simulink model "Bibliotheque"  (R2015a)
settings: Solver=ode45  StartTime=0.0  StopTime=10.0  RelTol=1e-3
undefined symbols (not defined in the file): B, D, dt, fv, gain_accelero, gain_effort_ext, gain_encodeur_moteur_rad, gain_intensite_moteur, gain_joy_X, gain_regle_mg, gain_tension_moteur, gain_vitesse_mm_s, gain_vitesse_tr_min, I, kprim, L, meq, National_Instruments, offset_effort_ext, offset_joy_X, offset_joy_Y, P, PCIe, r, sigbuilder_block, vecteur_de_tensions, vecteur_des_distances, Vsat
libraries: sldrtlib x35, simulink x4
settings Model: CovSFcnEnable=off  Creator=user  LastModifiedBy=ASUS
settings DataIOCC: SignalLoggingSaveFormat=ModelDataLogs
settings OptimizationCC: ExpressionDepthLimit=2147483647
settings DebuggingCC: UnderspecifiedInitializationDetection=Classic  MergeDetectMultiDrivingBlocksExec=none  SolverPrmCheckMsg=warning  FcnCallInpInsideContextMsg=EnableAllAsWarning  StateNameClashWarn=warning
settings GRTTargetCC: CombineOutputUpdateFcns=off  GRTInterface=on

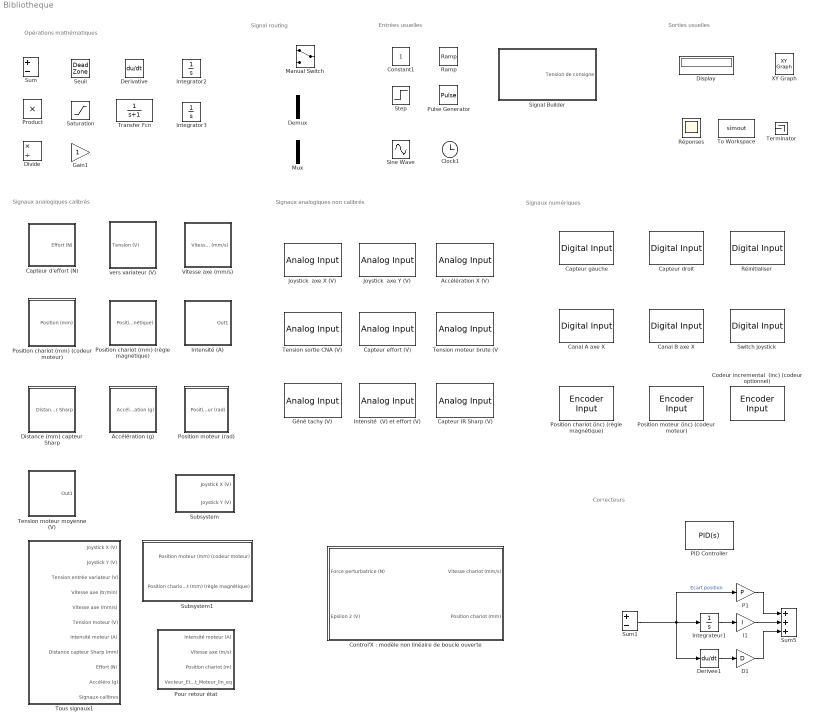
== system Bibliotheque ==
  note: Signaux numériques
  note: Signaux analogiques non calibrés
  note: Signaux analogiques calibrés
  note: Opérations mathématiques
  note: Signal routing
  note: Sorties usuelles
  note: Entrées usuelles
  note: Correcteurs
  Accélération (g) : Subsystem
      mask Display: image(imread('carte.jpg'))
  Accélération X (V) : sldrtlib/Analog Input  SampleTime=dt  MaxMissedTicks=10  ShowMissedTicks=off  YieldWhenWaiting=off  DrvName=National_Instruments/PCIe-6321  DrvAddress=4294967295  DrvOptions=[0 0 0 2 2 2 0]  Channels=15  RangeMode=1  VoltRange=1  DataType=1
      settings: AttributesFormatString=National Instruments\nPCIe-6321 [auto]
  Canal A axe X : sldrtlib/Digital Input  SampleTime=dt  MaxMissedTicks=10  ShowMissedTicks=off  YieldWhenWaiting=on  DrvName=National_Instruments/PCIe-6321  DrvAddress=4294967295  DrvOptions=[0 0 0 2 2 2 0]  Channels=5  BitMode=1  DataType=1
      settings: AttributesFormatString=National Instruments\nPCIe-6321 [auto]
  Canal B axe X : sldrtlib/Digital Input  SampleTime=dt  MaxMissedTicks=10  ShowMissedTicks=off  YieldWhenWaiting=on  DrvName=National_Instruments/PCIe-6321  DrvAddress=4294967295  DrvOptions=[0 0 0 2 2 2 0]  Channels=4  BitMode=1  DataType=1
      settings: AttributesFormatString=National Instruments\nPCIe-6321 [auto]
  Capteur IR Sharp (V) : sldrtlib/Analog Input  SampleTime=dt  MaxMissedTicks=10  ShowMissedTicks=off  YieldWhenWaiting=off  DrvName=National_Instruments/PCIe-6321  DrvAddress=4294967295  DrvOptions=[0 0 0 2 2 2 0]  Channels=7  RangeMode=1  VoltRange=1  DataType=1
      settings: AttributesFormatString=National Instruments\nPCIe-6321 [auto]
  Capteur d'effort (N) : Subsystem
      mask Display: image(imread('carte.jpg'))
  Capteur droit : sldrtlib/Digital Input  SampleTime=dt  MaxMissedTicks=10  ShowMissedTicks=off  YieldWhenWaiting=on  DrvName=National_Instruments/PCIe-6321  DrvAddress=4294967295  DrvOptions=[0 0 0 2 2 2 0]  Channels=2  BitMode=1  DataType=1
      settings: AttributesFormatString=National Instruments\nPCIe-6321 [auto]
  Capteur effort (V) : sldrtlib/Analog Input  SampleTime=dt  MaxMissedTicks=10  ShowMissedTicks=off  YieldWhenWaiting=off  DrvName=National_Instruments/PCIe-6321  DrvAddress=4294967295  DrvOptions=[0 0 0 2 2 2 0]  Channels=14  RangeMode=1  VoltRange=1  DataType=1
      settings: AttributesFormatString=National Instruments\nPCIe-6321 [auto]
  Capteur gauche : sldrtlib/Digital Input  SampleTime=dt  MaxMissedTicks=10  ShowMissedTicks=off  YieldWhenWaiting=on  DrvName=National_Instruments/PCIe-6321  DrvAddress=4294967295  DrvOptions=[0 0 0 2 2 2 0]  Channels=3  BitMode=1  DataType=1
      settings: AttributesFormatString=National Instruments\nPCIe-6321 [auto]
  Clock1 : Clock
  Codeur incremental  (inc) (codeur optionnel) : sldrtlib/Encoder Input  SampleTime=dt  MaxMissedTicks=10  ShowMissedTicks=off  YieldWhenWaiting=off  DrvName=National_Instruments/PCIe-6321  DrvAddress=4294967295  DrvOptions=[0 0 0 2 2 2 2]  Channels=4  QuadMode=3  IndexPulse=1  InputFilter=Inf  DataType=1
      settings: AttributesFormatString=National Instruments\nPCIe-6321 [auto]
  Constant1 : Constant  SampleTime=dt
  "Control'X : modèle non linéaire de boucle ouverte" : Subsystem
      mask Display:
      | image('Control''X.jpg')
      | port_label('output', 1, 'v (mm/s)')
      | port_label('output', 2, 'x (mm)')
      | port_label('input', 1, 'Fext (N)')
      | port_label('input', 2, 'eps2 (V)')
  D1 : Gain  Gain=D
  Demux : Demux  Outputs=2
  Derivative : Derivative
  Derivee1 : Derivative
  Display : Display
  Distance (mm) capteur Sharp : Subsystem
      mask Display: image(imread('carte.jpg'))
  Divide : Product  Inputs=*/
  Gain1 : Gain
  Géné tachy (V) : sldrtlib/Analog Input  SampleTime=dt  MaxMissedTicks=10  ShowMissedTicks=off  YieldWhenWaiting=off  DrvName=National_Instruments/PCIe-6321  DrvAddress=4294967295  DrvOptions=[0 0 0 2 2 2 0]  Channels=4  RangeMode=1  VoltRange=1  DataType=1
      settings: AttributesFormatString=National Instruments\nPCIe-6321 [auto]
  I1 : Gain  Gain=I
  Integrateur1 : Integrator
  Integrator2 : Integrator
  Integrator3 : Integrator  InitialConditionSource=external
  Intensité  (V) et effort (V) : sldrtlib/Analog Input  SampleTime=dt  MaxMissedTicks=10  ShowMissedTicks=off  YieldWhenWaiting=off  DrvName=National_Instruments/PCIe-6321  DrvAddress=4294967295  DrvOptions=[0 0 0 2 2 2 0]  Channels=[6,14]  RangeMode=1  VoltRange=1  DataType=1
      settings: AttributesFormatString=National Instruments\nPCIe-6321 [auto]
  Intensité (A) : Subsystem
      mask Display: image(imread('carte.jpg'))
  Joystick  axe X (V) : sldrtlib/Analog Input  SampleTime=dt  MaxMissedTicks=10  ShowMissedTicks=off  YieldWhenWaiting=off  DrvName=National_Instruments/PCIe-6321  DrvAddress=4294967295  DrvOptions=[0 0 0 2 2 2 0]  Channels=1  RangeMode=1  VoltRange=1  DataType=1
      settings: AttributesFormatString=National Instruments\nPCIe-6321 [auto]
  Joystick  axe Y (V) : sldrtlib/Analog Input  SampleTime=dt  MaxMissedTicks=10  ShowMissedTicks=off  YieldWhenWaiting=off  DrvName=National_Instruments/PCIe-6321  DrvAddress=4294967295  DrvOptions=[0 0 0 2 2 2 0]  Channels=2  RangeMode=1  VoltRange=1  DataType=1
      settings: AttributesFormatString=National Instruments\nPCIe-6321 [auto]
  Manual Switch : ManualSwitch
  Mux : Mux  Inputs=2
  P1 : Gain  Gain=P
  PID Controller : simulink/Continuous/PID Controller  Controller=PID  TimeDomain=Continuous-time  SampleTime=-1  IntegratorMethod=Forward Euler  FilterMethod=Forward Euler  Form=Parallel  UseFilter=on  ControllerParametersSource=internal  P=1  I=1  D=0  N=100  InitialConditionSource=internal  InitialConditionForIntegrator=0  InitialConditionForFilter=0  ExternalReset=none  LimitOutput=off  UpperSaturationLimit=inf  LowerSaturationLimit=-inf  LinearizeAsGain=off  AntiWindupMode=none  Kb=1  TrackingMode=off  Kt=1  PParamMin=[]  PParamMax=[]  IParamMin=[]  IParamMax=[]  DParamMin=[]  DParamMax=[]  NParamMin=[]  NParamMax=[]  KbParamMin=[]  KbParamMax=[]  KtParamMin=[]  KtParamMax=[]  POutMin=[]  POutMax=[]  IOutMin=[]  IOutMax=[]  DOutMin=[]  DOutMax=[]  NOutMin=[]  NOutMax=[]  KbOutMin=[]  KbOutMax=[]  KtOutMin=[]  KtOutMax=[]  IntegratorOutMin=[]  IntegratorOutMax=[]  FilterOutMin=[]  FilterOutMax=[]  SumOutMin=[]  SumOutMax=[]  SumI1OutMin=[]  SumI1OutMax=[]  SumI2OutMin=[]  SumI2OutMax=[]  SumI3OutMin=[]  SumI3OutMax=[]  SumDOutMin=[]  SumDOutMax=[]  SaturationOutMin=[]  SaturationOutMax=[]  IntegratorContinuousStateAttributes=''  IntegratorStateMustResolveToSignalObject=off  IntegratorRTWStateStorageClass=Auto  FilterContinuousStateAttributes=''  FilterStateMustResolveToSignalObject=off  FilterRTWStateStorageClass=Auto  DifferentiatorICPrevScaledInput=0  DifferentiatorOutMin=[]  DifferentiatorOutMax=[]
  Position chariot (inc) (règle magnétique) : sldrtlib/Encoder Input  SampleTime=dt  MaxMissedTicks=10  ShowMissedTicks=off  YieldWhenWaiting=off  DrvName=National_Instruments/PCIe-6321  DrvAddress=4294967295  DrvOptions=[0 0 0 2 2 2 0]  Channels=2  QuadMode=3  IndexPulse=1  InputFilter=Inf  DataType=1
      settings: AttributesFormatString=National Instruments\nPCIe-6321 [auto]
  Position chariot (mm) (codeur moteur) : Subsystem
      mask Display: image(imread('carte.jpg'))
  Position chariot (mm) (règle magnétique) : Subsystem
      mask Display: image(imread('carte.jpg'))
  Position moteur (inc) (codeur moteur) : sldrtlib/Encoder Input  SampleTime=dt  MaxMissedTicks=10  ShowMissedTicks=off  YieldWhenWaiting=off  DrvName=National_Instruments/PCIe-6321  DrvAddress=4294967295  DrvOptions=[0 0 0 2 2 2 0]  Channels=1  QuadMode=3  IndexPulse=1  InputFilter=Inf  DataType=1
      settings: AttributesFormatString=National Instruments\nPCIe-6321 [auto]
  Position moteur (rad) : Subsystem
      mask Display: image(imread('carte.jpg'))
  Pour retour état : Subsystem
      mask Display:
      | %image(imread('carte.jpg'))
      | port_label('output', 1, 'Intensité moteur (A)')
      | port_label('output', 2, 'Vitesse axe (m/s)')
      | port_label('output', 3, 'Position chariot(m)')
      | port_label('output', 4, 'Bus Tous Signaux')
  Product : Product  RndMeth=Zero
  Pulse Generator : DiscretePulseGenerator  PulseType=Time based  Amplitude=100  Period=5  PulseWidth=50
  Ramp : simulink/Sources/Ramp  slope=1  start=0  X0=0
  Réinitialiser : sldrtlib/Digital Input  SampleTime=dt  MaxMissedTicks=10  ShowMissedTicks=off  YieldWhenWaiting=on  DrvName=National_Instruments/PCIe-6321  DrvAddress=4294967295  DrvOptions=[0 0 0 2 2 2 0]  Channels=1  BitMode=1  DataType=1
      settings: AttributesFormatString=National Instruments\nPCIe-6321 [auto]
  Réponses : Scope
      settings: ShowLegends=on  TimeRange=10  YMin=-20  YMax=120  SaveName=y2  MaxDataPoints=10001
  Saturation : Saturate
  Seuil : DeadZone  SaturateOnIntegerOverflow=on
  Signal Builder : Subsystem  Tag=STV Subsys  LoadFcn=sigbuilder_block('load');  StartFcn=sigbuilder_block('start');  StopFcn=sigbuilder_block('stop');  ClipboardFcn=sigbuilder_block('clipboard');  mask(Sigbuilder block){}
      mask help: Create and generate interchangeable groups of signals whose waveforms are piecewise linear.
      mask init:
      | if ~strcmp(get_param(bdroot(gcbh),'SimulationStatus'),'stopped') tuvar = sigbuilder_block('maskInit'); end
      settings: CopyFcn=sigbuilder_block('copy');  DeleteFcn=sigbuilder_block('delete');  ModelCloseFcn=sigbuilder_block('modelClose');  PreSaveFcn=sigbuilder_block('preSave');  PauseFcn=sigbuilder_block('pause')  ContinueFcn=sigbuilder_block('continue')  NameChangeFcn=sigbuilder_block('namechange');  OpenFcn=sigbuilder_block('open',[141 150 550.5 399.75 ]);  CloseFcn=sigbuilder_block('close');
      mask Display: plot(0,0,100,100,[10,10,40,40,10],[80,20,20,80,80],[40,10],[50,50], [40,27,10],[65,72,56],[40,25,25,10],[28,28,43,43]);
  Sine Wave : Sin  Amplitude=5  Frequency=2*pi
  Step : Step  SampleTime=0
  Subsystem : Subsystem
  Subsystem1 : Subsystem
  Sum : Sum  Inputs=+-
  Sum1 : Sum  Inputs=+-
  Sum5 : Sum  Inputs=+++
  Switch joystick : sldrtlib/Digital Input  SampleTime=dt  MaxMissedTicks=10  ShowMissedTicks=off  YieldWhenWaiting=on  DrvName=National_Instruments/PCIe-6321  DrvAddress=4294967295  DrvOptions=[0 0 0 2 2 2 0]  Channels=6  BitMode=1  DataType=1
      settings: AttributesFormatString=National Instruments\nPCIe-6321 [auto]
  "Tension moteur brute (V " : sldrtlib/Analog Input  SampleTime=dt  MaxMissedTicks=10  ShowMissedTicks=off  YieldWhenWaiting=off  DrvName=National_Instruments/PCIe-6321  DrvAddress=4294967295  DrvOptions=[0 0 0 2 2 2 0]  Channels=5  RangeMode=1  VoltRange=1  DataType=1
      settings: AttributesFormatString=National Instruments\nPCIe-6321 [auto]
  Tension moteur moyenne (V) : Subsystem
      mask Display: image(imread('carte.jpg'))
  Tension sortie CNA (V) : sldrtlib/Analog Input  SampleTime=dt  MaxMissedTicks=10  ShowMissedTicks=off  YieldWhenWaiting=off  DrvName=National_Instruments/PCIe-6321  DrvAddress=4294967295  DrvOptions=[0 0 0 2 2 2 0]  Channels=3  RangeMode=1  VoltRange=1  DataType=1
      settings: AttributesFormatString=National Instruments\nPCIe-6321 [auto]
  Terminator : Terminator
  To Workspace : ToWorkspace  VariableName=simout  SampleTime=-1
  Tous signaux1 : Subsystem
      mask Display:
      | %image(imread('carte.jpg'))
      | port_label('output', 1, 'Joystick Axe X (V)')
      | port_label('output', 2, 'Joystick Axe Y (V)')
      | port_label('output', 3, 'Tension entrée variateur (V)')
      | port_label('output', 4, 'Vitesse moteur (tr/min)')
      | port_label('output', 5, 'Vitesse axe (mm/s)')
      | port_label('output', 6, 'Tension moteur (V)')
      | port_label('output', 7, 'Intensité moteur (A)')
      | port_label('output', 8, 'Distance capteur Sharp (mm)')
      | port_label('output', 9, 'Effort extérieur (N)')
      | port_label('output', 10, 'Accélération axe (g)')
      | port_label('output', 11, 'Bus Tous Signaux')
  Transfer Fcn : TransferFcn  Denominator=[1 1]
  Vitesse axe (mm/s) : Subsystem
      mask Display: image(imread('carte.jpg'))
  XY Graph : simulink/Sinks/XY Graph  xmin=-1  xmax=1  ymin=-1  ymax=1  st=-1
  vers variateur (V) : Subsystem
      mask Display: image(imread('carte.jpg'))
  wires:
  Sum1/1 -> Integrateur1/1, Derivee1/1, P1/1  "Ecart position"
  Integrateur1/1 -> I1/1
  Derivee1/1 -> D1/1
  I1/1 -> Sum5/2
  D1/1 -> Sum5/3
  P1/1 -> Sum5/1

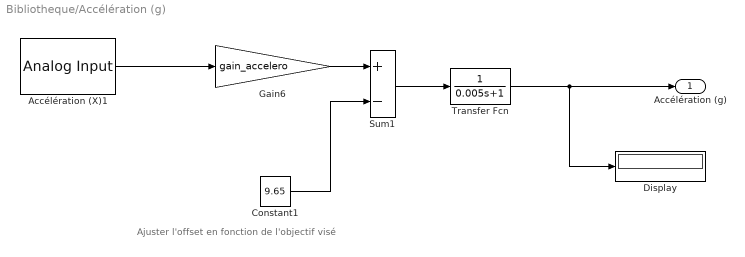
== system Bibliotheque/Accélération (g) ==
  note: Ajuster l'offset en fonction de l'objectif visé
  Accélération (X)1 : sldrtlib/Analog Input  SampleTime=dt  MaxMissedTicks=10  ShowMissedTicks=off  YieldWhenWaiting=off  DrvName=National_Instruments/PCIe-6321  DrvAddress=4294967295  DrvOptions=[0 0 0 2 2 2 0]  Channels=15  RangeMode=1  VoltRange=1  DataType=1
      settings: AttributesFormatString=National Instruments\nPCIe-6321 [auto]
  Constant1 : Constant  Value=9.65  SampleTime=dt
  Display : Display
  Gain6 : Gain  Gain=gain_accelero
  Sum1 : Sum  Inputs=+-
  Transfer Fcn : TransferFcn  Denominator=[0.005 1]
  Accélération (g) : Outport
  wires:
  Accélération (X)1/1 -> Gain6/1
  Gain6/1 -> Sum1/1
  Constant1/1 -> Sum1/2
  Transfer Fcn/1 -> Display/1, Accélération (g)/1
  Sum1/1 -> Transfer Fcn/1

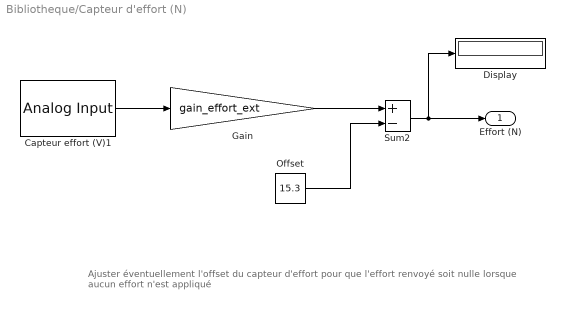
== system Bibliotheque/Capteur d'effort (N) ==
  note: Ajuster éventuellement l'offset du capteur d'effort pour que
      | l'effort renvoyé soit nulle lorsque aucun effort n'est appliqué
  Capteur effort (V)1 : sldrtlib/Analog Input  SampleTime=dt  MaxMissedTicks=10  ShowMissedTicks=off  YieldWhenWaiting=off  DrvName=National_Instruments/PCIe-6321  DrvAddress=4294967295  DrvOptions=[0 0 0 2 2 2 0]  Channels=14  RangeMode=1  VoltRange=1  DataType=1
      settings: AttributesFormatString=National Instruments\nPCIe-6321 [auto]
  Display : Display
  Gain : Gain  Gain=gain_effort_ext
  Offset : Constant  Value=15.3
  Sum2 : Sum  Inputs=+-
  Effort (N) : Outport
  wires:
  Gain/1 -> Sum2/1
  Capteur effort (V)1/1 -> Gain/1
  Sum2/1 -> Display/1, Effort (N)/1
  Offset/1 -> Sum2/2

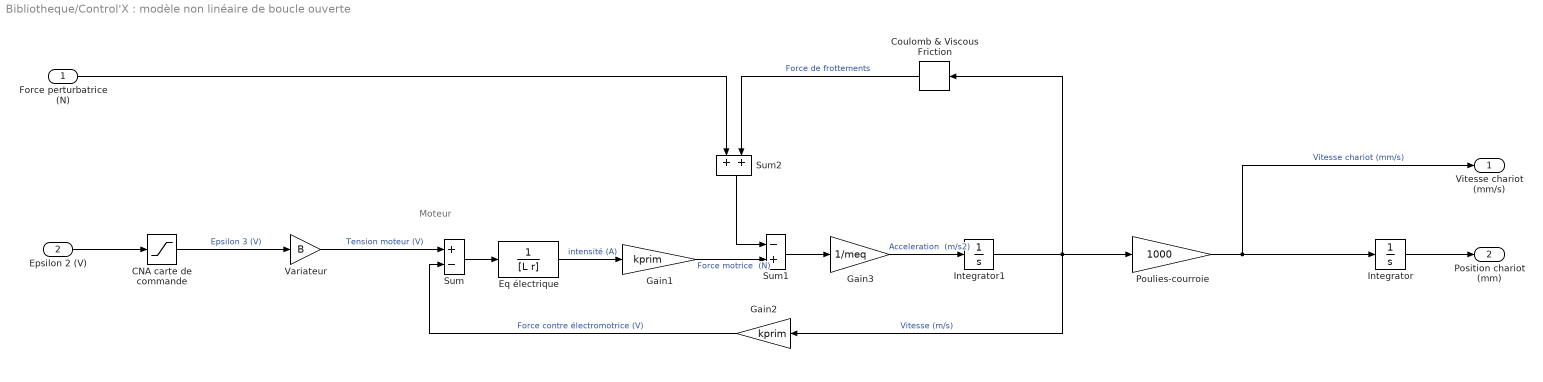
== system Bibliotheque/Control'X : modèle non linéaire de boucle ouverte ==
  note: Moteur
  Force perturbatrice (N) : Inport
  Epsilon 2 (V) : Inport  Port=2
  CNA carte de commande : Saturate  UpperLimit=Vsat  LowerLimit=-Vsat
  Coulomb & Viscous Friction : simulink/Discontinuities/Coulomb & Viscous Friction  offset=Ffrott  gain=fv
  Eq électrique : TransferFcn  Denominator=[L r]
  Gain1 : Gain  Gain=kprim
  Gain2 : Gain  Gain=kprim
  Gain3 : Gain  Gain=1/meq
  Integrator : Integrator
  Integrator1 : Integrator
  Poulies-courroie : Gain  Gain=1000
  Sum : Sum  Inputs=+-
  Sum1 : Sum  Inputs=-+
  Sum2 : Sum
  Variateur : Gain  Gain=B
  Vitesse chariot (mm/s) : Outport
  Position chariot (mm) : Outport  Port=2
  wires:
  Coulomb & Viscous Friction/1 -> Sum2/2  "Force de frottements"
  Epsilon 2 (V)/1 -> CNA carte de commande/1
  CNA carte de commande/1 -> Variateur/1  "Epsilon 3 (V)"
  Eq électrique/1 -> Gain1/1  "intensité (A)"
  Variateur/1 -> Sum/1  "Tension moteur (V)"
  Integrator1/1 -> Poulies-courroie/1, Coulomb & Viscous Friction/1, Gain2/1  "Vitesse (m/s)"
  Sum/1 -> Eq électrique/1
  Gain2/1 -> Sum/2  "Force contre électromotrice (V)"
  Gain1/1 -> Sum1/2  "Force motrice  (N)"
  Sum1/1 -> Gain3/1
  Poulies-courroie/1 -> Vitesse chariot (mm/s)/1, Integrator/1  "Vitesse chariot (mm/s)"
  Sum2/1 -> Sum1/1
  Integrator/1 -> Position chariot (mm)/1
  Gain3/1 -> Integrator1/1  "Acceleration  (m/s2)"
  Force perturbatrice (N)/1 -> Sum2/1

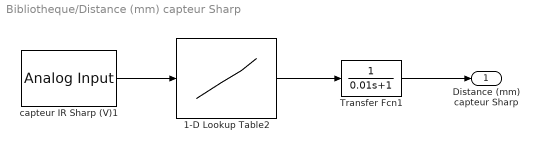
== system Bibliotheque/Distance (mm) capteur Sharp ==
  1-D Lookup Table2 : Lookup_n-D  NumberOfTableDimensions=1  BreakpointsForDimension1=vecteur_de_tensions  Table=vecteur_des_distances  ExtrapMethod=Clip  UseLastTableValue=on  InternalRulePriority=Speed  RndMeth=Simplest  InputSameDT=on
  Transfer Fcn1 : TransferFcn  Denominator=[0.01 1]
  capteur IR Sharp (V)1 : sldrtlib/Analog Input  SampleTime=dt  MaxMissedTicks=10  ShowMissedTicks=off  YieldWhenWaiting=off  DrvName=National_Instruments/PCIe-6321  DrvAddress=4294967295  DrvOptions=[0 0 0 2 2 2 0]  Channels=7  RangeMode=1  VoltRange=1  DataType=1
      settings: AttributesFormatString=National Instruments\nPCIe-6321 [auto]
  Distance (mm) capteur Sharp : Outport
  wires:
  capteur IR Sharp (V)1/1 -> 1-D Lookup Table2/1
  1-D Lookup Table2/1 -> Transfer Fcn1/1
  Transfer Fcn1/1 -> Distance (mm) capteur Sharp/1

== system Bibliotheque/Intensité (A) ==
  Intensité  (V) et effort (V) : sldrtlib/Analog Input  SampleTime=dt  MaxMissedTicks=10  ShowMissedTicks=off  YieldWhenWaiting=off  DrvName=National_Instruments/PCIe-6321  DrvAddress=4294967295  DrvOptions=[0 0 0 2 2 2 0]  Channels=[6]  RangeMode=1  VoltRange=1  DataType=1
      settings: AttributesFormatString=National Instruments\nPCIe-6321 [auto]
  gain_intensite_moteur : Gain  Gain=gain_intensite_moteur
  Out1 : Outport
  wires:
  gain_intensite_moteur/1 -> Out1/1
  Intensité  (V) et effort (V)/1 -> gain_intensite_moteur/1

== system Bibliotheque/Position chariot (mm) (codeur moteur) ==
  Adaptateur1 : Gain  Gain=D
  Codeur incremental : sldrtlib/Encoder Input  SampleTime=dt  MaxMissedTicks=10  ShowMissedTicks=off  YieldWhenWaiting=off  DrvName=National_Instruments/PCIe-6321  DrvAddress=4294967295  DrvOptions=[0 0 0 2 2 2 0]  Channels=1  QuadMode=3  IndexPulse=1  InputFilter=Inf  DataType=1
      settings: AttributesFormatString=National Instruments\nPCIe-6321 [auto]
  Position (mm) : Outport
  wires:
  Codeur incremental/1 -> Adaptateur1/1  "Position réelle (inc)"
  Adaptateur1/1 -> Position (mm)/1  "Position reelle (mm)"

== system Bibliotheque/Position chariot (mm) (règle magnétique) ==
  note: Dans cette boite, l'option "reset" ou "none" du champ "Rest input function"
      | permet de valider ou non le canal Z (top 0 situé à mi-course) de la règle magnétique.
      |
      | Il s'agit d'une remise à 0 automatique du compteur au passage du top 0.
  Position chariot (inc) : sldrtlib/Encoder Input  SampleTime=dt  MaxMissedTicks=10  ShowMissedTicks=off  YieldWhenWaiting=off  DrvName=National_Instruments/PCIe-6321  DrvAddress=4294967295  DrvOptions=[0 0 0 2 2 2 0]  Channels=2  QuadMode=3  IndexPulse=1  InputFilter=Inf  DataType=1
      settings: AttributesFormatString=National Instruments\nPCIe-6321 [auto]
  gain_regle_mg_mm : Gain  Gain=gain_regle_mg
  Position chariot (mm) (règle magnétique) : Outport
  wires:
  gain_regle_mg_mm/1 -> Position chariot (mm) (règle magnétique)/1
  Position chariot (inc)/1 -> gain_regle_mg_mm/1

== system Bibliotheque/Position moteur (rad) ==
  Position moteur (inc) : sldrtlib/Encoder Input  SampleTime=dt  MaxMissedTicks=10  ShowMissedTicks=off  YieldWhenWaiting=off  DrvName=National_Instruments/PCIe-6321  DrvAddress=4294967295  DrvOptions=[0 0 0 2 2 2 0]  Channels=1  QuadMode=3  IndexPulse=2  InputFilter=Inf  DataType=1
      settings: AttributesFormatString=National Instruments\nPCIe-6321 [auto]
  gain_encodeur_moteur_rad : Gain  Gain=gain_encodeur_moteur_rad
  Position moteur (rad) : Outport
  wires:
  gain_encodeur_moteur_rad/1 -> Position moteur (rad)/1
  Position moteur (inc)/1 -> gain_encodeur_moteur_rad/1

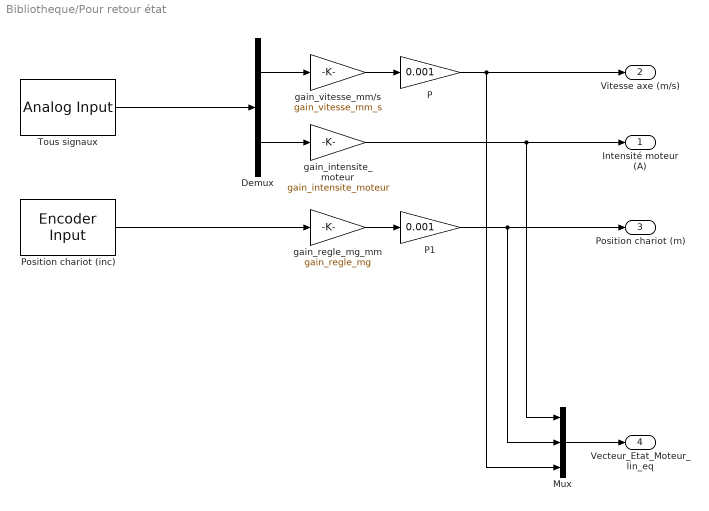
== system Bibliotheque/Pour retour état ==
  Demux : Demux  Outputs=2
  Mux : Mux  Inputs=3
  P : Gain  Gain=0.001
  P1 : Gain  Gain=0.001
  Position chariot (inc) : sldrtlib/Encoder Input  SampleTime=dt  MaxMissedTicks=10  ShowMissedTicks=off  YieldWhenWaiting=off  DrvName=National_Instruments/PCIe-6321  DrvAddress=4294967295  DrvOptions=[0 0 0 2 2 2 0]  Channels=2  QuadMode=3  IndexPulse=2  InputFilter=Inf  DataType=1
      settings: AttributesFormatString=National Instruments\nPCIe-6321 [auto]
  Tous signaux : sldrtlib/Analog Input  SampleTime=dt  MaxMissedTicks=10  ShowMissedTicks=off  YieldWhenWaiting=off  DrvName=National_Instruments/PCIe-6321  DrvAddress=4294967295  DrvOptions=[0 0 0 2 2 2 0]  Channels=[4 6]  RangeMode=1  VoltRange=1  DataType=1
      settings: AttributesFormatString=National Instruments\nPCIe-6321 [auto]
  gain_intensite_moteur : Gain  Gain=gain_intensite_moteur
  gain_regle_mg_mm : Gain  Gain=gain_regle_mg
  gain_vitesse_mm/s : Gain  Gain=gain_vitesse_mm_s
  Intensité moteur (A) : Outport
  Vitesse axe (m/s) : Outport  Port=2
  Position chariot (m) : Outport  Port=3
  Vecteur_Etat_Moteur_lin_eq : Outport  Port=4
  wires:
  Tous signaux/1 -> Demux/1
  gain_vitesse_mm/s/1 -> P/1
  gain_intensite_moteur/1 -> Mux/1, Intensité moteur (A)/1
  Demux/1 -> gain_vitesse_mm/s/1
  Demux/2 -> gain_intensite_moteur/1
  Position chariot (inc)/1 -> gain_regle_mg_mm/1
  Mux/1 -> Vecteur_Etat_Moteur_lin_eq/1
  P/1 -> Mux/3, Vitesse axe (m/s)/1
  P1/1 -> Mux/2, Position chariot (m)/1
  gain_regle_mg_mm/1 -> P1/1

== system Bibliotheque/Signal Builder ==
  Demux : Demux  Tag=STV Demux  Outputs=1
  FromWs : FromWorkspace  Tag=STV FromWs  VariableName=tuvar  SampleTime=0
      SigBuilderData=|
      | common.afterFinalStr = 'Extrapolate'
      | common.sampleTime = 0
      | dataSet.timeRange = [0 5]
      | dataSet.name = 'Group 1'
      | sbobj.Groups.Name = 'Group 1'
      | sbobj.Groups.Signals.Name = 'Tension de consigne'
      | sbobj.Groups.Signals.XData = [0 1 1 2 2 3 3 4 4 5]
      | sbobj.Groups.Signals.YData = [0 0 5 5 0 0 -5 -5 0 0]
  Tension de consigne : Outport  Tag=STV Outport
  wires:
  Demux/1 -> Tension de consigne/1
  FromWs/1 -> Demux/1

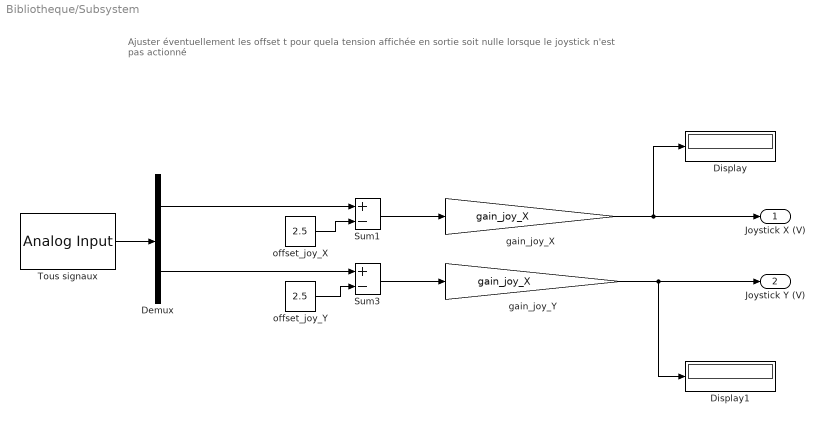
== system Bibliotheque/Subsystem ==
  note: Ajuster éventuellement les offset t pour quela tension affichée
      | en sortie soit nulle lorsque le joystick n'est pas actionné
  Demux : Demux  Outputs=2
  Display : Display
  Display1 : Display
  Sum1 : Sum  Inputs=+-
  Sum3 : Sum  Inputs=+-
  Tous signaux : sldrtlib/Analog Input  SampleTime=dt  MaxMissedTicks=10  ShowMissedTicks=off  YieldWhenWaiting=off  DrvName=National_Instruments/PCIe-6321  DrvAddress=4294967295  DrvOptions=[0 0 0 2 2 2 0]  Channels=[1 2]  RangeMode=1  VoltRange=1  DataType=1
      settings: AttributesFormatString=National Instruments\nPCIe-6321 [auto]
  gain_joy_X : Gain  Gain=gain_joy_X
  gain_joy_Y : Gain  Gain=gain_joy_X
  offset_joy_X : Constant  Value=2.5
  offset_joy_Y : Constant  Value=2.5
  Joystick X (V) : Outport
  Joystick Y (V) : Outport  Port=2
  wires:
  Demux/2 -> Sum3/1
  gain_joy_Y/1 -> Joystick Y (V)/1, Display1/1
  Demux/1 -> Sum1/1
  Sum1/1 -> gain_joy_X/1
  Sum3/1 -> gain_joy_Y/1
  Tous signaux/1 -> Demux/1
  gain_joy_X/1 -> Joystick X (V)/1, Display/1
  offset_joy_Y/1 -> Sum3/2
  offset_joy_X/1 -> Sum1/2

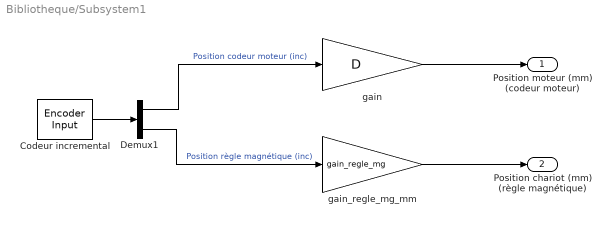
== system Bibliotheque/Subsystem1 ==
  Codeur incremental : sldrtlib/Encoder Input  SampleTime=dt  MaxMissedTicks=10  ShowMissedTicks=off  YieldWhenWaiting=off  DrvName=National_Instruments/PCIe-6321  DrvAddress=4294967295  DrvOptions=[0 0 0 2 2 2 2]  Channels=[1,2]  QuadMode=3  IndexPulse=1  InputFilter=Inf  DataType=1
      settings: AttributesFormatString=National Instruments\nPCIe-6321 [auto]
  Demux1 : Demux  Outputs=2
  gain : Gain  Gain=D
  gain_regle_mg_mm : Gain  Gain=gain_regle_mg
  Position moteur (mm) (codeur moteur) : Outport
  Position chariot (mm) (règle magnétique) : Outport  Port=2
  wires:
  gain/1 -> Position moteur (mm) (codeur moteur)/1
  Codeur incremental/1 -> Demux1/1
  Demux1/1 -> gain/1  "Position codeur moteur (inc)"
  Demux1/2 -> gain_regle_mg_mm/1  "Position règle magnétique (inc)"
  gain_regle_mg_mm/1 -> Position chariot (mm) (règle magnétique)/1

== system Bibliotheque/Tension moteur moyenne (V) ==
  P : Gain  Gain=gain_tension_moteur
  "Tension moteur brute (V " : sldrtlib/Analog Input  SampleTime=dt  MaxMissedTicks=10  ShowMissedTicks=off  YieldWhenWaiting=off  DrvName=National_Instruments/PCIe-6321  DrvAddress=4294967295  DrvOptions=[0 0 0 2 2 2 0]  Channels=5  RangeMode=1  VoltRange=1  DataType=1
      settings: AttributesFormatString=National Instruments\nPCIe-6321 [auto]
  Out1 : Outport
  wires:
  "Tension moteur brute (V "/1 -> P/1
  P/1 -> Out1/1

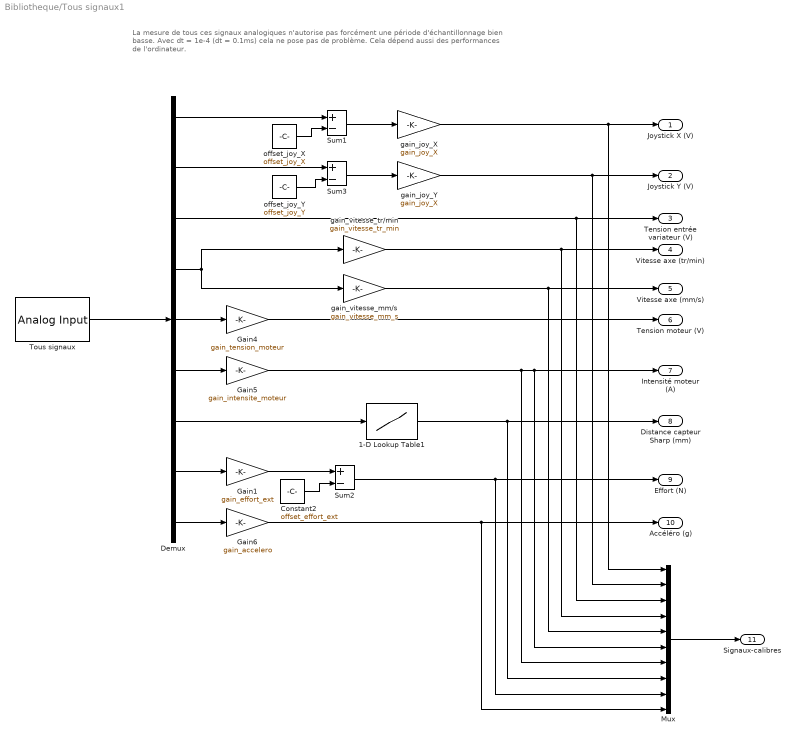
== system Bibliotheque/Tous signaux1 ==
  note: La mesure de tous ces signaux analogiques n'autorise pas forcément une période d'échantillonnage bien basse.
      | Avec dt = 1e-4 (dt = 0.1ms) cela ne pose pas de problème. Cela dépend aussi des performances de l'ordinateur.
  1-D Lookup Table1 : Lookup_n-D  NumberOfTableDimensions=1  BreakpointsForDimension1=vecteur_de_tensions  Table=vecteur_des_distances  ExtrapMethod=Clip  UseLastTableValue=on  InternalRulePriority=Speed  RndMeth=Simplest  InputSameDT=on
  Constant2 : Constant  Value=offset_effort_ext
  Demux : Demux  Outputs=9
  Gain1 : Gain  Gain=gain_effort_ext
  Gain4 : Gain  Gain=gain_tension_moteur
  Gain5 : Gain  Gain=gain_intensite_moteur
  Gain6 : Gain  Gain=gain_accelero
  Mux : Mux  Inputs=10
  Sum1 : Sum  Inputs=+-
  Sum2 : Sum  Inputs=+-
  Sum3 : Sum  Inputs=+-
  Tous signaux : sldrtlib/Analog Input  SampleTime=dt  MaxMissedTicks=10  ShowMissedTicks=off  YieldWhenWaiting=off  DrvName=National_Instruments/PCIe-6321  DrvAddress=4294967295  DrvOptions=[0 0 0 2 2 2 0]  Channels=[1 2 3 4 5 6 7 14 15]  RangeMode=1  VoltRange=1  DataType=1
      settings: AttributesFormatString=National Instruments\nPCIe-6321 [auto]
  gain_joy_X : Gain  Gain=gain_joy_X
  gain_joy_Y : Gain  Gain=gain_joy_X
  gain_vitesse_mm/s : Gain  Gain=gain_vitesse_mm_s
  gain_vitesse_tr/min : Gain  Gain=gain_vitesse_tr_min
  offset_joy_X : Constant  Value=offset_joy_X
  offset_joy_Y : Constant  Value=offset_joy_Y
  Joystick X (V) : Outport
  Joystick Y (V) : Outport  Port=2
  Tension entrée variateur (V) : Outport  Port=3
  Vitesse axe (tr/min) : Outport  Port=4
  Vitesse axe (mm/s) : Outport  Port=5
  Tension moteur (V) : Outport  Port=6
  Intensité moteur (A) : Outport  Port=7
  Distance capteur Sharp (mm) : Outport  Port=8
  Effort (N) : Outport  Port=9
  Accéléro (g) : Outport  Port=10
  Signaux-calibres : Outport  Port=11
  wires:
  Gain6/1 -> Mux/10, Accéléro (g)/1
  Demux/9 -> Gain6/1
  1-D Lookup Table1/1 -> Mux/8, Distance capteur Sharp (mm)/1
  Demux/7 -> 1-D Lookup Table1/1
  Gain5/1 -> Mux/7, Mux/6, Intensité moteur (A)/1
  Demux/6 -> Gain5/1
  Gain4/1 -> Tension moteur (V)/1
  Demux/5 -> Gain4/1
  gain_vitesse_mm/s/1 -> Mux/5, Vitesse axe (mm/s)/1
  gain_vitesse_tr/min/1 -> Mux/4, Vitesse axe (tr/min)/1
  Demux/4 -> gain_vitesse_tr/min/1, gain_vitesse_mm/s/1
  Demux/3 -> Mux/3, Tension entrée variateur (V)/1
  Sum3/1 -> gain_joy_Y/1
  Sum1/1 -> gain_joy_X/1
  offset_joy_Y/1 -> Sum3/2
  offset_joy_X/1 -> Sum1/2
  Demux/2 -> Sum3/1
  Demux/1 -> Sum1/1
  Demux/8 -> Gain1/1
  Tous signaux/1 -> Demux/1
  Gain1/1 -> Sum2/1
  Sum2/1 -> Mux/9, Effort (N)/1
  Constant2/1 -> Sum2/2
  gain_joy_X/1 -> Mux/1, Joystick X (V)/1
  gain_joy_Y/1 -> Mux/2, Joystick Y (V)/1
  Mux/1 -> Signaux-calibres/1

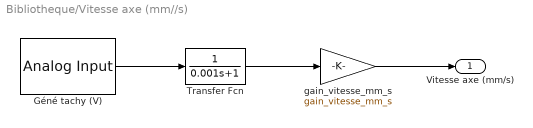
== system Bibliotheque/Vitesse axe (mm//s) ==
  Géné tachy (V) : sldrtlib/Analog Input  SampleTime=dt  MaxMissedTicks=10  ShowMissedTicks=off  YieldWhenWaiting=off  DrvName=National_Instruments/PCIe-6321  DrvAddress=4294967295  DrvOptions=[0 0 0 2 2 2 0]  Channels=4  RangeMode=1  VoltRange=1  DataType=1
      settings: AttributesFormatString=National Instruments\nPCIe-6321 [auto]
  Transfer Fcn : TransferFcn  Denominator=[0.001 1]
  gain_vitesse_mm_s : Gain  Gain=gain_vitesse_mm_s
  Vitesse axe (mm/s) : Outport
  wires:
  gain_vitesse_mm_s/1 -> Vitesse axe (mm/s)/1
  Transfer Fcn/1 -> gain_vitesse_mm_s/1
  Géné tachy (V)/1 -> Transfer Fcn/1

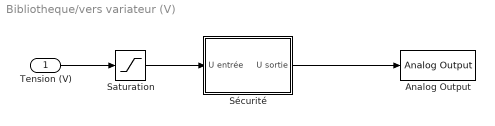
== system Bibliotheque/vers variateur (V) ==
  Tension (V) : Inport
  Analog Output : sldrtlib/Analog Output  SampleTime=dt  MaxMissedTicks=10  ShowMissedTicks=off  YieldWhenWaiting=off  DrvName=National_Instruments/PCIe-6321  DrvAddress=4294967295  DrvOptions=[0 0 0 2 2 2 0]  Channels=1  RangeMode=1  VoltRange=1  InitialValue=[]  FinalValue=0
      settings: AttributesFormatString=National Instruments\nPCIe-6321 [auto]
  Saturation : Saturate  UpperLimit=10  LowerLimit=-10
  Sécurité : Subsystem
  wires:
  Sécurité/1(U sortie) -> Analog Output/1
  Saturation/1 -> Sécurité/1(U entrée)
  Tension (V)/1 -> Saturation/1

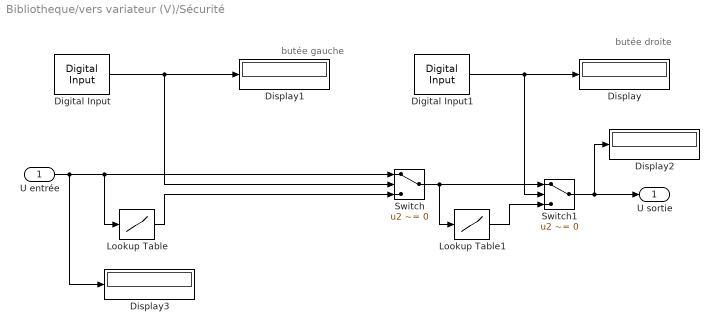
== system Bibliotheque/vers variateur (V)/Sécurité ==
  note: butée gauche
  note: butée droite
  U entrée : Inport
  Digital Input : sldrtlib/Digital Input  SampleTime=dt  MaxMissedTicks=10  ShowMissedTicks=off  YieldWhenWaiting=off  DrvName=National_Instruments/PCIe-6321  DrvAddress=4294967295  DrvOptions=[0 0 0 2 2 2 0]  Channels=3  BitMode=1  DataType=9
      settings: AttributesFormatString=National Instruments\nPCIe-6321 [auto]
  Digital Input1 : sldrtlib/Digital Input  SampleTime=dt  MaxMissedTicks=10  ShowMissedTicks=off  YieldWhenWaiting=off  DrvName=National_Instruments/PCIe-6321  DrvAddress=4294967295  DrvOptions=[0 0 0 2 2 2 0]  Channels=2  BitMode=1  DataType=9
      settings: AttributesFormatString=National Instruments\nPCIe-6321 [auto]
  Display{,1..3} (4 alike) : Display
      Display settings: Decimation=3
      Display2 settings: Decimation=3
      Display3 settings: Decimation=3
  Lookup Table : Lookup  InputValues=[-Vsat 0 Vsat]  Table=[0 0 Vsat]
  Lookup Table1 : Lookup  InputValues=[-Vsat 0 Vsat]  Table=[-Vsat 0 0]
  Switch : Switch  Criteria=u2 ~= 0
  Switch1 : Switch  Criteria=u2 ~= 0
  U sortie : Outport
  wires:
  U entrée/1 -> Lookup Table/1, Switch/1, Display3/1
  Digital Input/1 -> Switch/2, Display1/1
  Lookup Table/1 -> Switch/3
  Switch/1 -> Switch1/1, Lookup Table1/1
  Digital Input1/1 -> Switch1/2, Display/1
  Lookup Table1/1 -> Switch1/3
  Switch1/1 -> U sortie/1, Display2/1
